simulink model "model"  (R2013b)
settings: Solver=ode45  StartTime=0.0  StopTime=40  FixedStep=0.01  RelTol=1e-3
values from neighbouring files (symbols this model uses):
  c = 0.01    [consts.mat]
  g = 9.81    [consts.mat]
  L = 1    [consts.mat]
  m = 0.05    [consts.mat]
  st = 0.01    [consts.mat]
libraries: simulink x1
settings Model: Creator=maen  LastModifiedBy=Nabeel Ahmad
settings SolverCC: AutoInsertRateTranBlk=on
settings DataIOCC: SignalLoggingSaveFormat=ModelDataLogs
settings OptimizationCC: ExpressionDepthLimit=2147483647
settings DebuggingCC: FcnCallInpInsideContextMsg=UseLocalSettings  StateNameClashWarn=warning
settings GRTTargetCC: CombineOutputUpdateFcns=off  GRTInterface=on

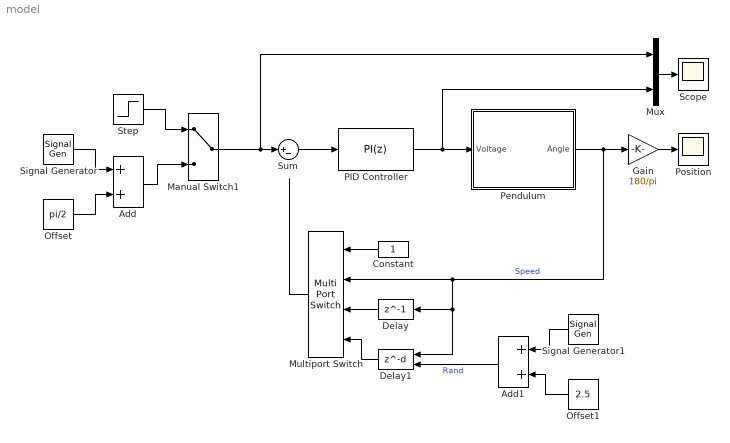
== system model ==
  Add : Sum
  Add1 : Sum  OutDataTypeStr=uint8
  Constant : Constant
  Delay : Delay  DelayLength=1  InitialCondition=0  SampleTime=st
  Delay1 : Delay  DelayLengthSource=Input port  InitialCondition=0  SampleTime=st
      settings: InputPortMap=u0,p1
  Gain : Gain  Gain=180/pi
  Manual Switch1 : ManualSwitch
  Multiport Switch : MultiPortSwitch
  Mux : Mux  Inputs=2
  Offset : Constant  Value=pi/2
  Offset1 : Constant  Value=2.5
  PID Controller : simulink/Continuous/PID Controller  Controller=PI  TimeDomain=Discrete-time  SampleTime=st  IntegratorMethod=Forward Euler  FilterMethod=Forward Euler  Form=Parallel  P=1  I=0  D=-6.78839610676139  N=58.2381885976492  InitialConditionSource=internal  InitialConditionForIntegrator=0  InitialConditionForFilter=0  ExternalReset=none  LimitOutput=off  UpperSaturationLimit=24  LowerSaturationLimit=0  LinearizeAsGain=on  AntiWindupMode=none  Kb=1  TrackingMode=off  Kt=1  PParamMin=[]  PParamMax=[]  IParamMin=[]  IParamMax=[]  DParamMin=[]  DParamMax=[]  NParamMin=[]  NParamMax=[]  KbParamMin=[]  KbParamMax=[]  KtParamMin=[]  KtParamMax=[]  POutMin=[]  POutMax=[]  IOutMin=[]  IOutMax=[]  DOutMin=[]  DOutMax=[]  NOutMin=[]  NOutMax=[]  KbOutMin=[]  KbOutMax=[]  KtOutMin=[]  KtOutMax=[]  IntegratorOutMin=[]  IntegratorOutMax=[]  FilterOutMin=[]  FilterOutMax=[]  SumOutMin=[]  SumOutMax=[]  SumI1OutMin=[]  SumI1OutMax=[]  SumI2OutMin=[]  SumI2OutMax=[]  SumI3OutMin=[]  SumI3OutMax=[]  SumDOutMin=[]  SumDOutMax=[]  SaturationOutMin=[]  SaturationOutMax=[]  IntegratorContinuousStateAttributes=''  IntegratorStateMustResolveToSignalObject=off  IntegratorRTWStateStorageClass=Auto  FilterContinuousStateAttributes=''  FilterStateMustResolveToSignalObject=off  FilterRTWStateStorageClass=Auto
  Pendulum : Subsystem
  Position : Scope
      settings: TimeRange=40  YMin=0  YMax=1200  SaveName=ScopeData2
  Scope : Scope
      settings: TimeRange=100  YMin=0  YMax=1.5
  Signal Generator : SignalGenerator  Amplitude=pi/4  Frequency=.2
  Signal Generator1 : SignalGenerator  Amplitude=2.5  Frequency=.05
  Step : Step  Time=2  After=.7  SampleTime=0
  Sum : Sum  Inputs=|+-
  wires:
  Mux/1 -> Scope/1
  PID Controller/1 -> Pendulum/1(Voltage), Mux/2
  Sum/1 -> PID Controller/1
  Manual Switch1/1 -> Mux/1, Sum/1
  Add/1 -> Manual Switch1/2
  Signal Generator/1 -> Add/1
  Offset/1 -> Add/2
  Step/1 -> Manual Switch1/1
  Delay/1 -> Multiport Switch/3
  Constant/1 -> Multiport Switch/1
  Delay1/1 -> Multiport Switch/4
  Pendulum/1(Angle) -> Gain/1, Delay1/1, Delay/1, Multiport Switch/2  "Speed"
  Multiport Switch/1 -> ?
  Offset1/1 -> Add1/2
  Signal Generator1/1 -> Add1/1
  Add1/1 -> Delay1/2  "Rand"
  Gain/1 -> Position/1

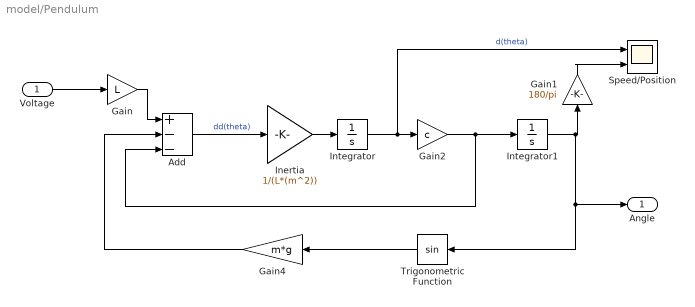
== system model/Pendulum ==
  Voltage : Inport
  Add : Sum  Inputs=+--
  Gain : Gain  Gain=L
  Gain1 : Gain  Gain=180/pi
  Gain2 : Gain  Gain=c
  Gain4 : Gain  Gain=m*g
  Inertia : Gain  Gain=1/(L*(m^2))
  Integrator : Integrator
  Integrator1 : Integrator
  Speed/Position : Scope  NumInputPorts=2
      settings: TimeRange=40  YMin=0~0  YMax=120~1200
  Trigonometric Function : Trigonometry
  Angle : Outport
  wires:
  Trigonometric Function/1 -> Gain4/1
  Inertia/1 -> Integrator/1
  Gain4/1 -> Add/2
  Integrator/1 -> Speed/Position/1, Gain2/1  "d(theta)"
  Voltage/1 -> Gain/1
  Add/1 -> Inertia/1  "dd(theta)"
  Gain/1 -> Add/1
  Integrator1/1 -> Angle/1, Trigonometric Function/1, Gain1/1
  Gain2/1 -> Add/3, Integrator1/1
  Gain1/1 -> Speed/Position/2
